simulink model "speedcontrolusingnormalinverter"  (R2022b)
settings: Solver=ode2  StartTime=0.0  StopTime=100  FixedStep=1e-5  RelTol=1e-3
libraries: spsIGBTDiodeLib x6, spsCurrentMeasurementLib x4, spsAsynchronousMachineSIUnitsLib x1, spsDCVoltageSourceLib x1, slpidlib x1, simulink x1, spsVoltageMeasurementLib x1, sps_lib x1
settings Model: SimulationMode=accelerator  Creator=bhuva  LastModifiedBy=bhuva

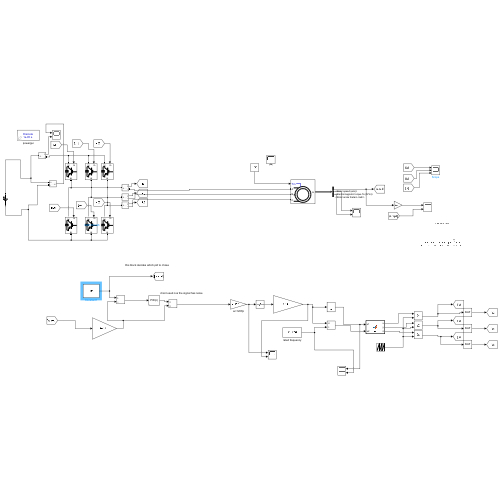
[thumbnail: Simulink's stored preview of the top-level diagram]
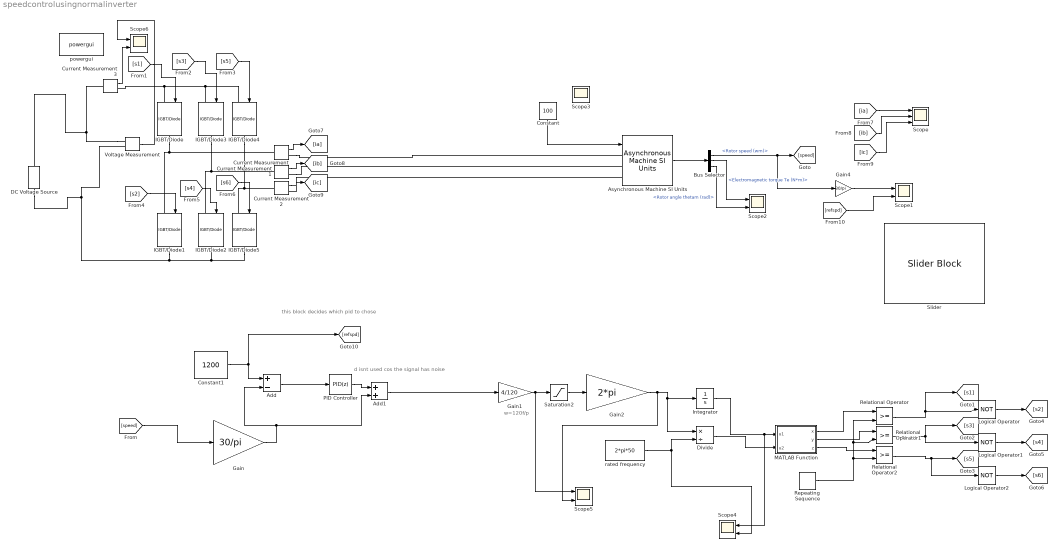
== system speedcontrolusingnormalinverter ==
  note: this block decides which pid to chose
  note: w=120f/p
  note: d isnt used cos the signal has noise
  Add : Sum  Inputs=+-
  Add1 : Sum
  Asynchronous Machine SI Units : spsAsynchronousMachineSIUnitsLib/Asynchronous Machine SI Units  RotorType=Squirrel-cage  PresetModel=No  MechanicalLoad=Torque Tm  ShowDetailedParameters=on  ReferenceFrame=Rotor  Units=SI  MeasurementBus=off  NominalParameters=[3.73e+04 400 50]  VoltageRatio=1  Stator=[0.09961 0.000867]  Rotor=[0.05837 0.000867]  Cage1=[0.4155 0.002066]  Cage2=[0.4168 0.0003495]  Lm=0.03039  Mechanical=[0.4 0.02187 2]  PolePairs=2  InitialConditions=[0 0 0 0 0 0 0 0]  SimulateSaturation=off  Saturation=[14.03593122, 27.81365428, 53.79336849, 72.68890987, 97.98006896, 148.6815601, 215.7428561, 302.9841135, 428.7778367 ; 230, 322, 414, 460, 506, 552, 598, 644, 690]  LoadFlowParameters=1492000  TsPowergui=0  TsBlock=1e-5  IterativeModel=Trapezoidal non iterative  IterativeDiscreteModel=Trapezoidal non iterative  Pmec=1.492e+006
  Bus Selector : BusSelector  OutputSignals=Mechanical.Rotor speed (wm),Mechanical.Electromagnetic torque Te (N*m),Mechanical.Rotor angle thetam (rad)
  Constant : Constant  Value=100
  Constant1 : Constant  Value=1200
  Current Measurement{,1..3} (4 alike) : spsCurrentMeasurementLib/Current Measurement  PhasorSimulation=off  OutputType=Complex  PSBequivalent=0
  DC Voltage Source : spsDCVoltageSourceLib/DC Voltage Source  Amplitude=500  Measurements=None
  Divide : Product  Inputs=*/
  Gain : Gain  Gain=30/pi
  Gain1 : Gain  Gain=4/120
  Gain2 : Gain  Gain=2*pi
  Gain4 : Gain  Gain=30/pi
  IGBT/Diode{,1..5} (6 alike) : spsIGBTDiodeLib/IGBT//Diode  Ron=1e-3  Rs=1e5  Cs=inf  Measurements=off
  Integrator : Integrator
  Logical Operator : Logic  Operator=NOT  AllPortsSameDT=off  OutDataTypeStr=boolean
  Logical Operator1 : Logic  Operator=NOT  AllPortsSameDT=off  OutDataTypeStr=boolean
  Logical Operator2 : Logic  Operator=NOT  AllPortsSameDT=off  OutDataTypeStr=boolean
  MATLAB Function : MATLAB Function  TreatAsAtomicUnit=on
  PID Controller : slpidlib/PID Controller  Controller=PID  Form=Parallel  TimeDomain=Discrete-time  UseExternalTs=off  SampleTime=1e-5  IntegratorMethod=Forward Euler  FilterMethod=Forward Euler  ControllerParametersSource=internal  P=0.75  I=5  UseKiTs=off  D=0.2  N=5000  UseFilter=on  TunerSelectOption=Frequency Response Based  ZeroCross=off  InitialConditionSource=internal  InitialConditionForIntegrator=0  InitialConditionForFilter=0  DifferentiatorICPrevScaledInput=0  ExternalReset=none  TrackingMode=off  Kt=1  LimitOutput=off  SatLimitsSource=internal  UpperSaturationLimit=inf  LowerSaturationLimit=-inf  LinearizeAsGain=on  AntiWindupMode=none  Kb=1  LimitIntegrator=off  UpperIntegratorSaturationLimit=inf  LowerIntegratorSaturationLimit=-inf  POutMin=[]  POutMax=[]  IOutMin=[]  IOutMax=[]  DOutMin=[]  DOutMax=[]  NOutMin=[]  NOutMax=[]  SumOutMin=[]  SumOutMax=[]  SaturationOutMin=[]  SaturationOutMax=[]  PParamMin=[]  PParamMax=[]  IParamMin=[]  IParamMax=[]  DParamMin=[]  DParamMax=[]  NParamMin=[]  NParamMax=[]  KbParamMin=[]  KbParamMax=[]  KtParamMin=[]  KtParamMax=[]  KbOutMin=[]  KbOutMax=[]  KtOutMin=[]  KtOutMax=[]  IntegratorOutMin=[]  IntegratorOutMax=[]  FilterOutMin=[]  FilterOutMax=[]  SumI1OutMin=[]  SumI1OutMax=[]  SumI2OutMin=[]  SumI2OutMax=[]  SumI3OutMin=[]  SumI3OutMax=[]  SumI4OutMin=[]  SumI4OutMax=[]  SumDOutMin=[]  SumDOutMax=[]  DifferentiatorOutMin=[]  DifferentiatorOutMax=[]  FilterDiffOutCoefMin=[]  FilterDiffOutCoefMax=[]  ReciprocalOutMin=[]  ReciprocalOutMax=[]  SumDenOutMin=[]  SumDenOutMax=[]  SumNumOutMin=[]  SumNumOutMax=[]  DivideOutMin=[]  DivideOutMax=[]  UdiffTsProdOutMin=[]  UdiffTsProdOutMax=[]  NTsProdOutMin=[]  NTsProdOutMax=[]  UintegralTsProdOutMin=[]  UintegralTsProdOutMax=[]  UngainTsProdOutMin=[]  UngainTsProdOutMax=[]  ClampingZeroOutDataTypeStr=Inherit: Inherit via back propagation  ClampingZeroOutMin=[]  ClampingZeroOutMax=[]  FilterDenConstantOutDataTypeStr=Inherit: Inherit via back propagation  FilterDenConstantOutMin=[]  FilterDenConstantOutMax=[]  PCopyOutDataTypeStr=Inherit: Inherit via back propagation  PCopyOutMin=[]  PCopyOutMax=[]  NCopyOutDataTypeStr=Inherit: Inherit via back propagation  NCopyOutMin=[]  NCopyOutMax=[]  IntegratorContinuousStateAttributes=''  IntegratorStateMustResolveToSignalObject=off  IntegratorRTWStateStorageClass=Auto  FilterContinuousStateAttributes=''  FilterStateMustResolveToSignalObject=off  FilterRTWStateStorageClass=Auto  ParallelPVariant=InternalParameters  IdealPVariant=Disabled  IVariant=InternalParameters  DVariant=InternalParameters  IntegratorVariant=Discrete  SatVariant=Disabled  AWVariant=Passthrough  PCopyVariant=Disabled  TRVariant=Disabled  FdbkBlocksVariant=Forward  IdealPFdbkVariant=Disabled  SatFdbkVariant=Disabled  DerivativeFilterVariant=ForwardEulerFilter  NVariant=InternalParameters  NCopyVariant=Disabled  FilterICVariant=InternalICsFilter  IntegratorICVariant=InternalICs  ExternalResetVariant=Disabled  TRSumVariant=Passthrough  SumFdbkVariant=Disabled  SumVariant=Sum_PID  TsampFilterVariant=InternalTs  TsampNgainVariant=Passthrough  TsampIntegralVariant=Passthrough  ExternalSaturationOutDataTypeStr=Inherit: Same as second input
  Relational Operator : RelationalOperator  OutDataTypeStr=boolean  InputSameDT=off
  Relational Operator1 : RelationalOperator  OutDataTypeStr=boolean  InputSameDT=off
  Relational Operator2 : RelationalOperator  OutDataTypeStr=boolean  InputSameDT=off
  Repeating Sequence : simulink/Sources/Repeating Sequence  rep_seq_t=[0 1 2]*(1/5000)  rep_seq_y=[-1 0 1]
  Saturation2 : Saturate  UpperLimit=50  LowerLimit=0
  Scope : Scope  NumInputPorts=3
  Scope{1..2,4..6} (5 alike) : Scope  NumInputPorts=2
  Scope3 : Scope
  Slider : SliderBlock  ScaleMax=1500
  Voltage Measurement : spsVoltageMeasurementLib/Voltage Measurement  PhasorSimulation=off  OutputType=Complex  PSBequivalent=0
  powergui : sps_lib/powergui  Priority=1  SimulationMode=Discrete  SampleTime=1e-5  frequency=60  Iterations=50  frequencyindice=0  Pbase=100e6  ErrMax=1e-4  UnitsV=kV  UnitsW=MW  buscounter=0  FunctionMessages=off  echomessages=off  EnableUseOfTLC=off  CurrentSourceSwitches=off  DisableSnubberDevices=off  DisableRonSwitches=off  DisableVfSwitches=off  DisplayEquations=off  AutomaticDiscreteSolvers=off  SolverType=Tustin  Interpol=off  ExternalGateDelay=off  methode=off  Ts=100  x0status=blocks  SPID=on  SwTol=0  HookPort=off  NonlinearTolerance=1e-4  nMaxIteration=100  ContinueOnMaxIteration=off  RestoreLinks=warning  ResistiveCurrentMeasurement=off  Frange=[0:2:500]  Ylog=off  Xlog=on  ShowGrid=off  save=off  variable=ZData  structure=0  ZoomFFT=off  StartTime=0.0  cycles=1  DisplayStyle=1  fundamental=60  FreqAxis=off  MaxFrequency=1000  frequencyindicesteady=1  RmsSteady=1  display=off
  rated frequency : Constant  Value=2*pi*50
  wires:
  Asynchronous Machine SI Units/1 -> Bus Selector/1
  Constant/1 -> Asynchronous Machine SI Units/1
  Constant1/1 -> Add/1, [refspd]
  Bus Selector/1 -> Gain4/1, [speed]  "<Rotor speed (wm)>"
  [speed] -> Gain/1
  Gain/1 -> Add/2, Add1/2
  Gain2/1 -> Scope5/2, Divide/1, Integrator/1
  rated frequency/1 -> Divide/2, Scope4/2
  [s1] -> IGBT/Diode/1
  [s3] -> IGBT/Diode3/1
  [s5] -> IGBT/Diode4/1
  Current Measurement2/1 -> [ic]
  Current Measurement1/1 -> [ib]
  Current Measurement/1 -> [ia]
  [ia] -> Scope/1
  [ib] -> Scope/2
  [ic] -> Scope/3
  [refspd] -> Scope1/2
  Gain4/1 -> Scope1/1
  Bus Selector/2 -> Scope2/1  "<Electromagnetic torque Te (N*m)>"
  Bus Selector/3 -> Scope2/2  "<Rotor angle thetam (rad)>"
  Gain1/1 -> Scope5/1, Saturation2/1
  [s2] -> IGBT/Diode1/1
  [s4] -> IGBT/Diode2/1
  [s6] -> IGBT/Diode5/1
  Integrator/1 -> Scope4/1, MATLAB Function/1(u1)
  MATLAB Function/3(z) -> Relational Operator2/1
  Logical Operator/1 -> [s2]
  Relational Operator/1 -> [s1], Logical Operator/1
  Repeating Sequence/1 -> Relational Operator1/2, Relational Operator/2, Relational Operator2/2
  Logical Operator2/1 -> [s6]
  MATLAB Function/2(y) -> Relational Operator1/1
  Divide/1 -> MATLAB Function/2(u2)
  Relational Operator2/1 -> Logical Operator2/1, [s5]
  MATLAB Function/1(x) -> Relational Operator/1
  Logical Operator1/1 -> [s4]
  Relational Operator1/1 -> [s3], Logical Operator1/1
  Saturation2/1 -> Gain2/1
  Current Measurement3/1 -> Scope6/2
  Voltage Measurement/1 -> Scope6/1
  Add/1 -> PID Controller/1
  PID Controller/1 -> Add1/1
  Add1/1 -> Gain1/1
  connections:
  IGBT/Diode3/RConn1 -- IGBT/Diode2/LConn1 -- Current Measurement1/LConn1
  IGBT/Diode1/RConn1 -- DC Voltage Source/LConn1 -- Voltage Measurement/LConn2 -- IGBT/Diode5/RConn1 -- IGBT/Diode2/RConn1
  IGBT/Diode/RConn1 -- IGBT/Diode1/LConn1 -- Current Measurement/LConn1
  IGBT/Diode4/RConn1 -- IGBT/Diode5/LConn1 -- Current Measurement2/LConn1
  Current Measurement3/RConn1 -- IGBT/Diode/LConn1 -- IGBT/Diode4/LConn1 -- IGBT/Diode3/LConn1
  Current Measurement/RConn1 -- Asynchronous Machine SI Units/LConn1
  Current Measurement2/RConn1 -- Asynchronous Machine SI Units/LConn3
  Current Measurement1/RConn1 -- Asynchronous Machine SI Units/LConn2
  Voltage Measurement/LConn1 -- DC Voltage Source/RConn1 -- Current Measurement3/LConn1

== matlab function speedcontrolusingnormalinverter/MATLAB Function ==
  data: x output; u1 input; y output; u2 input; z output
function [x,y,z] = fcn(u1,u2)

x = u2*sin(u1);
y = u2*sin(u1-(2*pi/3));
z = u2*sin(u1+(2*pi/3));
